simulink model "AFCSModel"  (R2025b)
settings: Solver=ode4  StartTime=0.0  StopTime=200  FixedStep=0.01  RelTol=1e-3  EnableMultiTasking=on
values from neighbouring files (symbols this model uses):
  AD = [0.05526	0.05526	0.05568	0.05804	0.06460	0.08210 ... (first row only)    [AirCraftData.m]
  Alpha0 = [0.143	0.143	0.122	-0.267	-0.627	0.120 ... (first row only)    [AirCraftData.m]
  alt = 1284.73    [Start.m]    (also in drl_simplified_dynamics.m)
  CA = 3.451    [AirCraftData.m]    (also in AircraftTrim.m)
  CDmin = [0.03799	0.03799	0.03799	0.03799	0.03904	0.04277 ... (first row only)    [AirCraftData.m]
  CLAlpha = [0.1012	0.1021	0.1033	0.1051	0.1079	0.0976 ... (first row only)    [AirCraftData.m]
  Clbt0 = [-0.00147	-0.00148	-0.00149	-0.00153	-0.00158	-0.00171 ... (first row only)    [AirCraftData.m]
  Clbtaf = [0	0	0	0	0	0;0	 0	0	0	0	0]    [AirCraftData.m]
  ClDelA = [-0.003110	-0.003065	-0.003040	-0.003036	-0.003052	-0.003088 ... (first row only)    [AirCraftData.m]
  CLDelE = [0.00653	0.00668	0.00690	0.00724	0.00772	0.00846 ... (first row only)    [AirCraftData.m]
  ClDelR = [0.000584	0.000605	0.000638	0.000686	0.000760	0.000877 ... (first row only)    [AirCraftData.m]
  CLDM = [0.244	0.244	0.244	0.244	0.244	0.244 ... (first row only)    [AirCraftData.m]
  Clp0 = [-0.5510 	-0.5610 	-0.5767 	-0.6005 	-0.6224 	-0.6763 ... (first row only)    [AirCraftData.m]
  ClpAf = [0,0,0,0,0,0;0,0,0,0,0,0]    [AirCraftData.m]
  Clr0 = [0.1308 	0.1339 	0.1383 	0.1474 	0.1601 	0.1738 ... (first row only)    [AirCraftData.m]
  ClrAf = [0,0,0,0,0,0;0,0,0,0,0,0]    [AirCraftData.m]
  Cm0 = [0.2014	0.2017	0.2034	0.2083	0.2207	0.2475 ... (first row only)    [AirCraftData.m]
  CmAfdot = [-11.5890 	-12.0169 	-12.7558 	-13.8010 	-15.2088 	-16.2278 ... (first row only)    [AirCraftData.m]
  CmCl = [-0.3454	-0.3441	-0.3427	-0.3412	-0.3396	-0.3379 ... (first row only)    [AirCraftData.m]
  CmDelE = [-0.03554	-0.03651	-0.03802	-0.04028	-0.04365	-0.04798 ... (first row only)    [AirCraftData.m]
  Cmq0 = [-42.0260 	-42.2665 	-42.9499 	-44.8315 	-45.5877 	-46.0842 ... (first row only)    [AirCraftData.m]
  CN1A0 = [0.0740	0.0662	0.0605	0.0552	0.0554 ... (first row only)    [AirCraftData.m]
  Cnbt0 = [0.00180	0.00183	0.00187	0.00192	0.00200	0.00207 ... (first row only)    [AirCraftData.m]
  Cnbtaf = [-0.000030 	-0.000031 	-0.000031 	-0.000032 	-0.000033 	-0.000035 ... (first row only)    [AirCraftData.m]
  CnDelA0 = [-0.000180	-0.000178	-0.000176	-0.000176	-0.000177	-0.000179 ... (first row only)    [AirCraftData.m]
  CnDelAAf = [0	 0	0	0	0	0;0	 0	0	0	0	0]    [AirCraftData.m]
  CnDelR = [-0.002214	-0.002274	-0.002367	-0.002505	-0.002712	-0.003039 ... (first row only)    [AirCraftData.m]
  Cnp0 = [0.0521 	0.0532 	0.0571 	0.0601 	0.0636 	0.0664 ... (first row only)    [AirCraftData.m]
  CnpAf = [0,0,0,0,0,0;0,0,0,0,0,0]    [AirCraftData.m]
  Cnr = [-0.1810 	-0.1832 	-0.1855 	-0.1892 	-0.1933 	-0.1973 ... (first row only)    [AirCraftData.m]
  Cxh_Slip = [0.0000, 0.0045, 0.0089, 0.0132, 0.0174 ... (first row only)    [AirCraftData.m]
  Cybeta0 = [-0.01783	-0.01790	-0.01804	-0.01824	-0.01851	-0.01884 ... (first row only)    [AirCraftData.m]
  Cybtaf = [0 0 0 0 0 0;0 0 0 0 0 0]    [AirCraftData.m]
  CyDelA = [0.000287	0.000295	0.000307	0.000325	0.000351	0.000394 ... (first row only)    [AirCraftData.m]
  CyDelR = [0.004946	0.005035	0.005316	0.005791	0.006458	0.007318 ... (first row only)    [AirCraftData.m]
  Cyh_Slip = [0.0000, -0.0248, -0.0519, -0.0813, -0.1130 ... (first row only)    [AirCraftData.m]
  ETA_data = [0.729 0.727 0.72 0.71 0.877 0.858 0.855 0.853 0.857 0.862 0.87 0.796 ... (330 elements, 11x5x6)]    [ETA_data.mat]
  eul_0 = [0/57.3 0/57.3 0/57.3]    [AircraftTrim.m]
  F = A(:, 1)    [drl_simplified_dynamics.m]    (also in func_DrawAircraftModel.m = [         1,  2,  3,  1;         1,  3,  4,  1;         1,  )
  flap = 0    [AircraftTrim.m]
  inertia = [  Ix      Iy     Iz  Ixz]    [AircraftTrim.m]
  Initi_Heading = 15.95*pi/180    (= 0.278380015693)    [Start.m]
  Initi_Lati = 32.6261    [Start.m]
  Initi_Longi = 103.5940    (= 103.594)    [Start.m]
  mass = 54000    [Start.m]    (also in drl_simplified_dynamics.m)
  op = evalin('base', 'op')    [drl_simplified_dynamics.m]
  q = func_GreatCircleForward(start_lat, start_lon, leg_bearing, local_s)    [system_model_update.m]
  r = r1 + r2    [drl_piecewise_reward.m]    (also in drl_reward_function.m)
  RNPAR_FlightPlan = JiuZhaiHuangLong_RNPAR_FlightPlan    [Manuscript_RNPAR_FlightPlan.m]
  Vab_0 = [Vt 0 0]    [AircraftTrim.m]
  Vt = 80    [Start.m]    (also in drl_simplified_dynamics.m; setup_afcs_system_model_test.m)
  wind_direction = 0    [Start.m]
  wind_type = 2    [Start.m]
  Wxyz_0 = [0 0 0]    [AircraftTrim.m]
  X = 1.06    [AircraftTrim.m]
  xme_0 = [0 0 -alt]    [AircraftTrim.m]
  Y = 1.177    [AircraftTrim.m]
undefined symbols (not defined in the file or in its folder): func_SystemModelMonitorBlock, Light, MIL, slselsubs, thrust_data
libraries: simulink_extras x4, aerolibatmos2 x3, aerolibconvert2 x3, aerolibwind2 x3, sharedutil x2, aerolibobsolete x1
(part 3 of 3)

== system AFCSModel/Plane&Actuator/PlaneModel/Aero Moment/Calculate pitch Moment M ==
  QS : Inport
  V alpha beta : Inport  Port=2
  delta_p : Inport  Port=3
  delta_a delta_e delta_r : Inport  Port=4
  p q r : Inport  Port=5
  Thrust : Inport  Port=6
  delta_flap : Inport  Port=7
  CA2 : Gain  Gain=CA*121.86
  CA4 : Gain  Gain=-2*(0.5208+0.5909)*9.8
  "Caculate CM " : Subsystem
  Calculate Delta_M : Subsystem
  Product4 : Product  RndMeth=Zero
  Selector13 : Selector  InputPortWidth=3  IndexOptions=Index vector (dialog)  Indices=[3]  OutputSizes=[(-2)]
  Selector2 : Selector  InputPortWidth=3  IndexOptions=Index vector (dialog)  Indices=[1 2 ]  OutputSizes=[(-2)]
  Selector3 : Selector  InputPortWidth=3  IndexOptions=Index vector (dialog)  Indices=[2]  OutputSizes=[(-2)]
  Selector9 : Selector  InputPortWidth=3  IndexOptions=Index vector (dialog)  Indices=[2]  OutputSizes=[(-2)]
  Sum4 : Sum  Inputs=++++
  disturb Moment : Gain  Gain=4*(92.12*12300+106.2*1075)*2*3.14159/60
  M : Outport
  wires:
  V alpha beta/1 -> Selector2/1
  delta_a delta_e delta_r/1 -> Selector3/1
  delta_p/1 -> "Caculate CM "/2(delta_p)
  p q r/1 -> Selector9/1, Selector13/1
  Selector9/1 -> "Caculate CM "/4(q)
  QS/1 -> CA2/1, Calculate Delta_M/2(Qs)
  CA2/1 -> Product4/1
  Product4/1 -> Sum4/1
  Thrust/1 -> CA4/1, Calculate Delta_M/3(Thrust)
  CA4/1 -> Sum4/2
  Selector13/1 -> disturb Moment/1
  disturb Moment/1 -> Sum4/4
  Sum4/1 -> M/1
  "Caculate CM "/1(Cm) -> Product4/2
  Selector3/1 -> "Caculate CM "/3(delta_e)
  Selector2/1 -> "Caculate CM "/1(" V Alpha"), Calculate Delta_M/1(" V Alpha")
  Calculate Delta_M/1(DelatM) -> Sum4/3
  delta_flap/1 -> "Caculate CM "/5(delta_flap)

== system AFCSModel/Plane&Actuator/PlaneModel/Display_Model/Normalize1 ==
  psi without normalizing : Inport
  Add6 : Sum
  Angle Conversion1 : aerolibconvert2/Angle Conversion  IU=rad  OU=deg
  Angle Conversion2 : aerolibconvert2/Angle Conversion  IU=deg  OU=rad
  Constant : Constant  Value=-360
  Constant2 : Constant  Value=360
  Constant4 : Constant  Value=360
  Math Function : Math  Operator=mod  SignedPower=on
  Math Function1 : Math  Operator=mod  SignedPower=on
  Sign : Signum
  Switch : Switch  Criteria=u2 > Threshold  SaturateOnIntegerOverflow=off  InputSameDT=off
  Switch1 : Switch  Criteria=u2 > Threshold  SaturateOnIntegerOverflow=off  InputSameDT=off
  Psi : Outport
  wires:
  Math Function/1 -> Switch1/3
  Constant2/1 -> Math Function1/2
  Math Function1/1 -> Switch1/1
  Angle Conversion1/1 -> Math Function/1, Math Function1/1, Sign/1
  Add6/1 -> Switch/3
  Switch/1 -> Angle Conversion2/1
  psi without normalizing/1 -> Angle Conversion1/1
  Constant/1 -> Math Function/2
  Constant4/1 -> Add6/2
  Sign/1 -> Switch1/2
  Switch1/1 -> Switch/1, Add6/1, Switch/2
  Angle Conversion2/1 -> Psi/1

== system AFCSModel/Plane&Actuator/PlaneModel/Display_Model/Position Caculate ==
  VE : Inport
  VN : Inport  Port=2
  H_in : Inport  Port=3
  Add{,1..3} (4 alike) : Sum
  Divide : Product  Inputs=/*
  Divide1 : Product  Inputs=*/
  Divide2 : Product  Inputs=*/
  Gain : Gain  Gain=180/pi
  Gain1 : Gain  Gain=180/pi
  Gain2 : Gain  Gain=pi/180
  Initial Latitudinal1 : Constant  Value=Initi_Longi
  Initial Latitudinal2 : Constant  Value=Initi_Lati
  Integrator : Integrator
  Integrator1 : Integrator
  Subsystem : Subsystem
  Trigonometric Function3 : Trigonometry  Operator=cos
  Latitude : Outport
  Longitude : Outport  Port=2
  wires:
  Integrator1/1 -> Add/1
  Integrator/1 -> Add1/1
  Gain2/1 -> Trigonometric Function3/1
  Gain1/1 -> Integrator/1
  Gain/1 -> Integrator1/1
  Add1/1 -> Longitude/1
  Initial Latitudinal1/1 -> Add1/2
  Divide1/1 -> Gain1/1
  Divide2/1 -> Divide1/1
  Trigonometric Function3/1 -> Divide1/2
  Add/1 -> Subsystem/1(L), Latitude/1, Gain2/1
  VN/1 -> Divide/2
  Initial Latitudinal2/1 -> Add/2
  Divide/1 -> Gain/1
  VE/1 -> Divide2/1
  Subsystem/1(RN) -> Add2/2
  H_in/1 -> Add3/2, Add2/1
  Add2/1 -> Divide2/2
  Subsystem/2(RM) -> Add3/1
  Add3/1 -> Divide/1

== system AFCSModel/Plane&Actuator/PlaneModel/Display_Model/TAS-IAS ==
  H : Inport
  V : Inport  Port=2
  TAS-EAS1 : Subsystem
  IAS : Outport
  wires:
  V/1 -> TAS-EAS1/1(TAS  (m/s))
  H/1 -> TAS-EAS1/2(Height  (m))
  TAS-EAS1/1(EAS (m/s)) -> IAS/1

== system AFCSModel/Plane&Actuator/PlaneModel/RusPlane/AV Alpha Beta ==
  udot vdot wdot : Inport
  Alpha dot : Fcn  Expr="(  - u[1]*u[6] + u[3]*u[4]  ) / ( u[4]*u[4]+ u[6]*u[6] )"
  Beta dot : Fcn  Expr="( u[7]*u[2]-u[5]*( (  u[1]*u[4] + u[2]*u[5] + u[3]*u[6] ) / u[7] ) ) / ( cos(u[9])*u[7]*u[7] )"
  Mux : Mux  Inputs=3
  Mux1 : Mux  Inputs=[3 3 3]
  Mux2 : Mux  Inputs=3
  V alpha beta : Integrator  InitialCondition=op.States(1).x
  V dot : Fcn  Expr="(  u[1]*u[4] + u[2]*u[5] + u[3]*u[6] ) / u[7]"
  "Vx " : Fcn  Expr=u[1]*cos(u[2])*cos(u[3])
  Vy1 : Fcn  Expr=u[1]*sin(u[2])*cos(u[3])
  Vz1 : Fcn  Expr=u[1]*sin(u[3])
  V alpha beta : Outport  InitialOutput=0
  u v w in : Outport  Port=2  InitialOutput=0
  wires:
  Mux2/1 -> V alpha beta/1
  V dot/1 -> Mux2/1
  Alpha dot/1 -> Mux2/2
  Beta dot/1 -> Mux2/3
  udot vdot wdot/1 -> Mux1/1
  Mux1/1 -> Alpha dot/1, V dot/1, Beta dot/1
  V alpha beta/1 -> V alpha beta/1, Mux1/3, "Vx "/1, Vz1/1, Vy1/1
  Mux/1 -> Mux1/2, u v w in/1
  "Vx "/1 -> Mux/1  "u"
  Vz1/1 -> Mux/2  "v"
  Vy1/1 -> Mux/3  "w"

== system AFCSModel/Plane&Actuator/PlaneModel/RusPlane/AV Alpha Beta_Trans ==
  V alpha beta input : Inport
  Alpha : Fcn  Expr=atan(u(3) / u(1))
  Beta : Fcn  Expr=asin(u(2) / sqrt(u(1)^2 + u(2)^2 + u(3)^2))
  Memory : Memory
  Mux : Mux  Inputs=3
  Mux2 : Mux  Inputs=3
  Sum3 : Sum  Inputs=+-
  V : Fcn  Expr=sqrt(u(1)^2 + u(2)^2 + u(3)^2)
  "Vx " : Fcn  Expr=u[1]*cos(u[2])*cos(u[3])
  Vy1 : Fcn  Expr=u[1]*sin(u[2])*cos(u[3])
  Vz1 : Fcn  Expr=u[1]*sin(u[3])
  Valphabeta : Outport
  wires:
  Vz1/1 -> Mux/2  "v"
  "Vx "/1 -> Mux/1  "u"
  Vy1/1 -> Mux/3  "w"
  V alpha beta input/1 -> Vy1/1, Vz1/1, "Vx "/1
  Mux/1 -> Sum3/1
  Mux2/1 -> Valphabeta/1
  Alpha/1 -> Mux2/2
  Beta/1 -> Mux2/3
  V/1 -> Mux2/1
  Sum3/1 -> V/1, Beta/1, Alpha/1
  [uvw_body] -> Memory/1
  Memory/1 -> Sum3/2

== system AFCSModel/Plane&Actuator/PlaneModel/RusPlane/Calculate DCM & Euler Angles ==
  "Wxyz " : Inport
  phi theta psi : Integrator  InitialCondition=[op.States(3).x(1) op.States(3).x(2) Initi_Heading]
  phidot psidot thetadot : Subsystem
  Euler : Outport
  wires:
  "Wxyz "/1 -> phidot psidot thetadot/1(Wx Wy Wz)
  phidot psidot thetadot/1(phidot thetadot psidot) -> phi theta psi/1
  phi theta psi/1 -> Euler/1, phidot psidot thetadot/2(phi theta psi)

== system AFCSModel/Plane&Actuator/PlaneModel/RusPlane/Subsystem ==
  Moment L M N : Inport
  pqr : Inport  Port=2
  inertia Ix Iy Iz Ixz : Inport  Port=3
  Beta dot : Fcn  Expr="( u[7]*u[3]+  u[1]*u[10] +  u[5]*u[6]*u[10]*(  u[8]-u[9]-u[7] )+  u[4]*u[5]*(  u[7]^2 - u[10]^2-u[7]*u[8]) ) / (u[7]*u[9]-u[10]^2)"
  Mux1 : Mux  Inputs=[3 3 4]
  Mux2 : Mux  Inputs=3
  p dot : Fcn  Expr=(u[1]*u[9] + u[3]*u[10] +u[4]*u[5]*u[10]* (u[7]+u[9]-u[8])-u[5]*u[6]*(u[9]^2+u[10]^2-u[8]*u[9])) / (u[7]*u[9]-u[10]^2)
  q dot : Fcn  Expr="( u[2]-u[4]*u[6]*(u[7]-u[9]) - u[10]*(u[4]^2-u[6]^2)  ) / u[8]"
  pdot qdot rdot : Outport
  wires:
  Mux1/1 -> Beta dot/1, p dot/1, q dot/1
  Mux2/1 -> pdot qdot rdot/1
  Beta dot/1 -> Mux2/3
  q dot/1 -> Mux2/2
  p dot/1 -> Mux2/1
  inertia Ix Iy Iz Ixz/1 -> Mux1/3
  pqr/1 -> Mux1/2
  Moment L M N/1 -> Mux1/1

== system AFCSModel/Plane&Actuator/PlaneModel/RusPlane/Subsystem1 ==
  "U V W " : Inport
  Euler phi theta psi : Inport  Port=2
  Mux1 : Mux  Inputs=[3 3 ]
  Mux2 : Mux  Inputs=3
  Xe dot : Fcn  Expr="u[1]*cos(u[5])*cos(u[6])  +   u[2]*(sin(u[4])*sin(u[5]) *cos(u[6])-cos(u[4])*sin(u[6]) )  +u[3]*(sin(u[4])*sin(u[6])+cos(u[4])*sin(u[5])*cos(u[6])  )"
  Ye dot : Fcn  Expr="u[1]*cos(u[5])*sin(u[6])  + u[2]*(sin(u[4])*sin(u[5])*sin(u[6]) + cos(u[4])*cos(u[6]) )  + u[3]*( cos(u[4])*sin(u[5])*sin(u[6])-sin(u[4])*cos(u[6]) )"
  Ze dot : Fcn  Expr="u[2]*sin(u[4])*cos(u[5])  + u[3]*cos(u[4])*cos(u[5]) -u[1]*sin(u[5])"
  Xedot Yedot Zedot : Outport
  wires:
  Xe dot/1 -> Mux2/1
  Ze dot/1 -> Mux2/3
  Mux2/1 -> Xedot Yedot Zedot/1
  "U V W "/1 -> Mux1/1
  Euler phi theta psi/1 -> Mux1/2
  Mux1/1 -> Xe dot/1, Ye dot/1, Ze dot/1
  Ye dot/1 -> Mux2/2

== system AFCSModel/Plane&Actuator/PlaneModel/Aero Force/Caculate Y/Cy_beta ==
  Ma : Inport
  alpha : Inport  Port=2
  delta_flap : Inport  Port=3
  Add1 : Sum
  Cy_beta0 : Lookup2D  RowIndex=[0 6/57.3]  ColumnIndex=Mach_table  Table=Cybeta0  SaturateOnIntegerOverflow=off  InputSameDT=off
  Cy_beta_alpha : Lookup2D  RowIndex=[0 6/57.3]  ColumnIndex=Mach_table  Table=Cybtaf  SaturateOnIntegerOverflow=off  InputSameDT=off
  Product5 : Product  RndMeth=Zero
  Cybeta : Outport
  wires:
  Cy_beta0/1 -> Add1/1
  Cy_beta_alpha/1 -> Product5/1
  Product5/1 -> Add1/2
  Ma/1 -> Cy_beta0/2, Cy_beta_alpha/2
  Add1/1 -> Cybeta/1
  alpha/1 -> Product5/2
  delta_flap/1 -> Cy_beta0/1, Cy_beta_alpha/1

== system AFCSModel/Plane&Actuator/PlaneModel/Aero Force/Calculate  Lift/Caculate CL ==
  Alpha : Inport
  delta_e : Inport  Port=2
  delta_flap : Inport  Port=3
  Alpha_0 : Lookup2D  RowIndex=[0 6/57.3]  ColumnIndex=Mach_table  Table=Alpha0  SaturateOnIntegerOverflow=off  InputSameDT=off
  Cl_alpha : Lookup2D  RowIndex=[0 6/57.3]  ColumnIndex=Mach_table  Table=CLAlpha  SaturateOnIntegerOverflow=off  InputSameDT=off
  Cl_alpha*alpha : Product  RndMeth=Zero
  Cl_delta_e*delta_e : Product  RndMeth=Zero
  Cldelta_e : Lookup2D  RowIndex=[0 6/57.3]  ColumnIndex=Mach_table  Table=CLDelE  SaturateOnIntegerOverflow=off  InputSameDT=off
  Constant : Constant  Value=4/57.3
  Subtract : Sum
  Subtract1 : Sum  Inputs=+-
  Subtract2 : Sum
  CL : Outport
  wires:
  Cldelta_e/1 -> Cl_delta_e*delta_e/1
  delta_e/1 -> Cl_delta_e*delta_e/2
  Constant/1 -> Subtract/1
  Alpha/1 -> Subtract/2
  [Ma] -> Alpha_0/2, Cldelta_e/2, Cl_alpha/2
  Subtract/1 -> Subtract1/1
  Alpha_0/1 -> Subtract1/2
  Cl_alpha/1 -> Cl_alpha*alpha/1
  Subtract1/1 -> Cl_alpha*alpha/2
  Cl_alpha*alpha/1 -> Subtract2/1
  Cl_delta_e*delta_e/1 -> Subtract2/2
  Subtract2/1 -> CL/1
  delta_flap/1 -> Cl_alpha/1, Alpha_0/1, Cldelta_e/1

== system AFCSModel/Plane&Actuator/PlaneModel/Aero Force/Calculate  Lift/SlipStream Strength B ==
  Thrust : Inport
  Qs : Inport  Port=2
  Divide : Product  Inputs=*/
  S : Gain  Gain=12.566
  B : Outport
  wires:
  S/1 -> Divide/2
  Qs/1 -> S/1
  Divide/1 -> B/1
  Thrust/1 -> Divide/1

== system AFCSModel/Plane&Actuator/PlaneModel/Aero Force/Calculate  Lift/alpha_w_deg ==
  In1 : Inport
  Constant : Constant  Value=4
  S3 : Gain  Gain=57.3
  Subtract : Sum
  Out1 : Outport
  wires:
  S3/1 -> Subtract/1
  Constant/1 -> Subtract/2
  In1/1 -> S3/1
  Subtract/1 -> Out1/1

== system AFCSModel/Plane&Actuator/PlaneModel/Aero Force/Calculate Drag/Caculate CD  ==
  " delta_flap" : Inport
  "  Alpha_w" : Inport  Port=2
  AD : Lookup2D  RowIndex=[0 6/57.3]  ColumnIndex=Mach_table  Table=AD  SaturateOnIntegerOverflow=off  InputSameDT=off
  Add : Sum
  Alpha0 : Lookup2D  RowIndex=[0 6/57.3]  ColumnIndex=Mach_table  Table=Alpha0  SaturateOnIntegerOverflow=off  InputSameDT=off
  CDmin : Lookup2D  RowIndex=[0 6/57.3]  ColumnIndex=Mach_table  Table=CDmin  SaturateOnIntegerOverflow=off  InputSameDT=off
  CLDM : Lookup2D  RowIndex=[0 6/57.3]  ColumnIndex=Mach_table  Table=CLDM  SaturateOnIntegerOverflow=off  InputSameDT=off
  Cl_alpha : Lookup2D  RowIndex=[0 6/57.3]  ColumnIndex=Mach_table  Table=CLAlpha  SaturateOnIntegerOverflow=off  InputSameDT=off
  Product : Product  RndMeth=Zero
  Product1 : Product  RndMeth=Zero
  Product2 : Product  RndMeth=Zero
  Subtract : Sum  Inputs=+-
  alpha_w-alpha0 : Sum  Inputs=-+
  CD : Outport
  wires:
  [Ma] -> Alpha0/2, CLDM/2, Cl_alpha/2, AD/2, CDmin/2
  CDmin/1 -> Add/1
  "  Alpha_w"/1 -> alpha_w-alpha0/2
  Alpha0/1 -> alpha_w-alpha0/1
  alpha_w-alpha0/1 -> Product/2
  Cl_alpha/1 -> Product/1
  Product/1 -> Subtract/1
  CLDM/1 -> Subtract/2
  Subtract/1 -> Product1/1, Product1/2
  AD/1 -> Product2/1
  Product1/1 -> Product2/2
  Product2/1 -> Add/2
  Add/1 -> CD/1
  " delta_flap"/1 -> CDmin/1, AD/1, Cl_alpha/1, Alpha0/1, CLDM/1

== system AFCSModel/Plane&Actuator/PlaneModel/Aero Force/Calculate Drag/SlipStream Strength B ==
  Thrust : Inport
  Qs : Inport  Port=2
  Divide : Product  Inputs=*/
  S : Gain  Gain=12.566
  B : Outport
  wires:
  S/1 -> Divide/2
  Qs/1 -> S/1
  Divide/1 -> B/1
  Thrust/1 -> Divide/1

== system AFCSModel/Plane&Actuator/PlaneModel/Aero Force/Calculate Drag/alpha_w_deg ==
  In1 : Inport
  Constant : Constant  Value=4
  S3 : Gain  Gain=57.3
  Subtract : Sum
  Out1 : Outport
  wires:
  S3/1 -> Subtract/1
  Constant/1 -> Subtract/2
  In1/1 -> S3/1
  Subtract/1 -> Out1/1

== system AFCSModel/Plane&Actuator/PlaneModel/Aero Moment/Calculate Roll Moment L/airdata ==
  V Alpha Beta : Inport
  delta_p : Inport  Port=2
  delta_flap : Inport  Port=3
  Add : Sum
  CN_alpha : Subsystem
  Cl_beta : Subsystem
  Cl_beta* : Sum
  Cl_delta_a : Lookup2D  RowIndex=[0 6/57.3]  ColumnIndex=Mach_table  Table=ClDelA  SaturateOnIntegerOverflow=off  InputSameDT=off
  Cl_delta_r : Lookup2D  RowIndex=[0 6/57.3]  ColumnIndex=Mach_table  Table=ClDelR  SaturateOnIntegerOverflow=off  InputSameDT=off
  Cl_delta_r* : Sum
  Cl_p : Subsystem
  Cl_r : Subsystem
  Cy_beta : Subsystem
  Cy_delta_r : Lookup2D  RowIndex=[0 6/57.3]  ColumnIndex=Mach_table  Table=CyDelR  SaturateOnIntegerOverflow=off  InputSameDT=off
  Gain : Gain  Gain=(Y-0.85)/38
  Gain1 : Gain  Gain=(Y-0.85)/38
  Mux2 : Mux  Inputs=5
  Selector1 : Selector  InputPortWidth=3  IndexOptions=Index vector (dialog)  Indices=[2]  OutputSizes=[(-2)]
  Selector12 : Selector  InputPortWidth=3  IndexOptions=Index vector (dialog)  Indices=[2]  OutputSizes=[(-2)]
  Cl_beta Cl_delta_a Cl_delta_r Cl_p Cl_r : Outport
  wires:
  [Ma] -> Cl_p/2(Ma), Cl_r/2(Ma), Cy_delta_r/2, Cl_delta_r/2, Cl_delta_a/2, Cy_beta/3(Ma), Cl_beta/1(Ma)
  Mux2/1 -> Cl_beta Cl_delta_a Cl_delta_r Cl_p Cl_r/1
  delta_p/1 -> CN_alpha/2(delta_p)
  V Alpha Beta/1 -> CN_alpha/1(V), Selector12/1, Selector1/1
  CN_alpha/1(Out1) -> Add/2
  Cy_beta/1(Cybeta) -> Gain/1
  Gain/1 -> Cl_beta*/2
  Add/1 -> Cl_beta*/1
  Cy_delta_r/1 -> Gain1/1
  Cl_delta_r/1 -> Cl_delta_r*/1
  Gain1/1 -> Cl_delta_r*/2
  Cl_beta*/1 -> Mux2/1
  Cl_delta_a/1 -> Mux2/2
  Cl_delta_r*/1 -> Mux2/3
  Cl_p/1(Cl_p) -> Mux2/4
  Cl_r/1(Cl_r) -> Mux2/5
  Selector12/1 -> Cl_p/1(alpha), Cl_r/1(alpha), Cl_r/3(delta_flap), Cy_beta/1(alpha)
  Cl_beta/1(C1beta) -> Add/1
  Selector1/1 -> Cl_beta/2(alpha)
  delta_flap/1 -> Cl_beta/3(delta_flap), Cy_beta/2(delta_flap), Cl_delta_a/1, Cl_delta_r/1, Cy_delta_r/1, Cl_p/3(delta_flap)

== system AFCSModel/Plane&Actuator/PlaneModel/Aero Moment/Calculate Yaw Moment N/aeroMoment coef ==
  V Alpha Beta : Inport
  delta_p : Inport  Port=2
  delta_flap : Inport  Port=3
  CN_alpha : Subsystem
  Cn_beta : Subsystem
  Cn_beta* : Sum  Inputs=+++
  Cn_delta_a1 : Subsystem
  Cn_delta_r : Lookup2D  RowIndex=[0 6/57.3]  ColumnIndex=Mach_table  Table=CnDelR  SaturateOnIntegerOverflow=off  InputSameDT=off
  Cn_delta_r* : Sum
  Cn_p : Subsystem
  Cn_r : Lookup2D  RowIndex=[0 6/57.3]  ColumnIndex=Mach_table  Table=Cnr  SaturateOnIntegerOverflow=off  InputSameDT=off
  Cy_beta : Subsystem
  Cy_delta_r : Lookup2D  RowIndex=[0 6/57.3]  ColumnIndex=Mach_table  Table=CyDelR  SaturateOnIntegerOverflow=off  InputSameDT=off
  Gain : Gain  Gain=(X-1.036514)/38
  Gain1 : Gain  Gain=(X-1.036514)/38
  Mux2 : Mux  Inputs=5
  Selector1 : Selector  InputPortWidth=3  IndexOptions=Index vector (dialog)  Indices=[1]  OutputSizes=[(-2)]
  Selector12 : Selector  InputPortWidth=3  IndexOptions=Index vector (dialog)  Indices=[2]  OutputSizes=[(-2)]
  Cn_beta Cn_delta_r Cl_delta_a Cn_p Cn_r : Outport
  wires:
  [Ma] -> Cn_p/2(Ma), Cn_r/2, Cn_delta_a1/2(Ma), Cy_delta_r/2, Cn_delta_r/2, Cy_beta/2(Ma), Cn_beta/2(Ma)
  Mux2/1 -> Cn_beta Cn_delta_r Cl_delta_a Cn_p Cn_r/1
  delta_p/1 -> CN_alpha/2(delta_p)
  V Alpha Beta/1 -> Selector12/1, Selector1/1
  Cn_beta*/1 -> Mux2/1
  CN_alpha/1(Out1) -> Cn_beta*/1
  Cn_beta/1(Cnbeta) -> Cn_beta*/2
  Cy_beta/1(Cybeta) -> Gain/1
  Gain/1 -> Cn_beta*/3
  Cy_delta_r/1 -> Gain1/1
  Gain1/1 -> Cn_delta_r*/2
  Cn_delta_r/1 -> Cn_delta_r*/1
  Cn_delta_r*/1 -> Mux2/2
  Cn_delta_a1/1(Cn_delta_a) -> Mux2/3
  Cn_p/1(Cn_p) -> Mux2/4
  Cn_r/1 -> Mux2/5
  Selector12/1 -> Cn_beta/1(alpha), Cy_beta/1(alpha), Cn_delta_a1/1(alpha), Cn_p/1(alpha)
  Selector1/1 -> CN_alpha/1(V)
  delta_flap/1 -> Cn_beta/3(delta_flap), Cy_beta/3(delta_flap), Cn_delta_r/1, Cy_delta_r/1, Cn_delta_a1/3(delta_flap), Cn_p/3(delta_flap), Cn_r/1

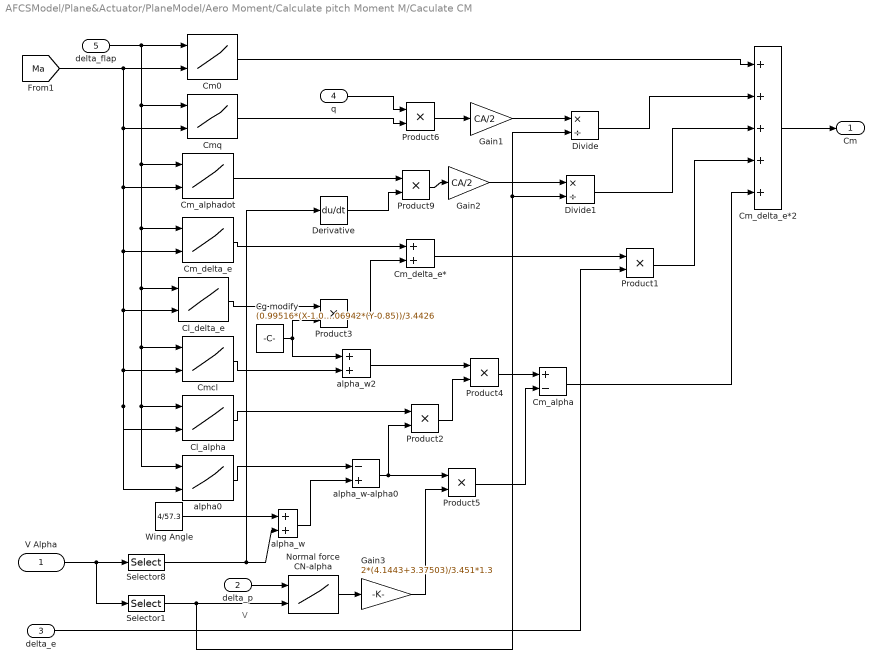
== system AFCSModel/Plane&Actuator/PlaneModel/Aero Moment/Calculate pitch Moment M/Caculate CM  ==
  note: V
  " V Alpha" : Inport
  delta_p : Inport  Port=2
  delta_e : Inport  Port=3
  q : Inport  Port=4
  delta_flap : Inport  Port=5
  Cg modify : Constant  Value=(0.99516*(X-1.036514)-0.06942*(Y-0.85))/3.4426
  Cl_alpha : Lookup2D  RowIndex=[0 6/57.3]  ColumnIndex=Mach_table  Table=CLAlpha  SaturateOnIntegerOverflow=off  InputSameDT=off
  Cl_delta_e : Lookup2D  RowIndex=[0 6/57.3]  ColumnIndex=Mach_table  Table=CLDelE  SaturateOnIntegerOverflow=off  InputSameDT=off
  Cm0 : Lookup2D  RowIndex=[0 6/57.3]  ColumnIndex=Mach_table  Table=Cm0  SaturateOnIntegerOverflow=off  InputSameDT=off
  Cm_alpha : Sum  Inputs=+-
  Cm_alphadot : Lookup2D  RowIndex=[0 6/57.3]  ColumnIndex=Mach_table  Table=CmAfdot  SaturateOnIntegerOverflow=off  InputSameDT=off
  Cm_delta_e : Lookup2D  RowIndex=[0 6/57.3]  ColumnIndex=Mach_table  Table=CmDelE  SaturateOnIntegerOverflow=off  InputSameDT=off
  Cm_delta_e* : Sum
  Cm_delta_e*2 : Sum  Inputs=+++++
  Cmcl : Lookup2D  RowIndex=[0 6/57.3]  ColumnIndex=Mach_table  Table=CmCl  SaturateOnIntegerOverflow=off  InputSameDT=off
  Cmq : Lookup2D  RowIndex=[0 6/57.3]  ColumnIndex=Mach_table  Table=Cmq0  SaturateOnIntegerOverflow=off  InputSameDT=off
  Derivative : Derivative
  Divide : Product  Inputs=*/
  Divide1 : Product  Inputs=*/
  Gain1 : Gain  Gain=CA/2
  Gain2 : Gain  Gain=CA/2
  Gain3 : Gain  Gain=2*(4.1443+3.37503)/3.451*1.3
  Normal force CN-alpha : Lookup2D  RowIndex=[0.4,0.7,0.85,1,1.04]  ColumnIndex=[50,75,100,150,175]  Table=CN1A0  SaturateOnIntegerOverflow=off  InputSameDT=off
  Product{1..6,9} (7 alike) : Product  RndMeth=Zero
  Selector1 : Selector  InputPortWidth=2  IndexOptions=Index vector (dialog)  Indices=[1]  OutputSizes=[(-2)]
  Selector8 : Selector  InputPortWidth=2  IndexOptions=Index vector (dialog)  Indices=[2]  OutputSizes=[(-2)]
  Wing Angle : Constant  Value=4/57.3
  alpha0 : Lookup2D  RowIndex=[0 6/57.3]  ColumnIndex=Mach_table  Table=Alpha0  SaturateOnIntegerOverflow=off  InputSameDT=off
  alpha_w : Sum
  alpha_w-alpha0 : Sum  Inputs=-+
  alpha_w2 : Sum
  Cm : Outport
  wires:
  [Ma] -> Cl_alpha/2, alpha0/2, Cmcl/2, Cl_delta_e/2, Cm_delta_e/2, Cm_alphadot/2, Cmq/2, Cm0/2
  Cm_delta_e*2/1 -> Cm/1
  " V Alpha"/1 -> Selector8/1, Selector1/1
  Wing Angle/1 -> alpha_w/1
  Selector8/1 -> alpha_w/2, Derivative/1
  alpha0/1 -> alpha_w-alpha0/1
  alpha_w/1 -> alpha_w-alpha0/2
  alpha_w-alpha0/1 -> Product2/2, Product5/1
  Cl_alpha/1 -> Product2/1
  Normal force CN-alpha/1 -> Gain3/1
  Selector1/1 -> Divide/2, Divide1/2, Normal force CN-alpha/2
  alpha_w2/1 -> Product4/1
  Cg modify/1 -> Product3/2, alpha_w2/1
  Cl_delta_e/1 -> Product3/1
  Cm_delta_e/1 -> Cm_delta_e*/1
  Product3/1 -> Cm_delta_e*/2
  Product2/1 -> Product4/2
  Product4/1 -> Cm_alpha/1
  Gain3/1 -> Product5/2
  Product5/1 -> Cm_alpha/2
  Cmcl/1 -> alpha_w2/2
  delta_e/1 -> Product1/2
  Cm_delta_e*/1 -> Product1/1
  q/1 -> Product6/1
  Cmq/1 -> Product6/2
  Product6/1 -> Gain1/1
  Gain1/1 -> Divide/1
  Gain2/1 -> Divide1/1
  Product9/1 -> Gain2/1
  Derivative/1 -> Product9/2
  Cm_alphadot/1 -> Product9/1
  Cm0/1 -> Cm_delta_e*2/1
  Divide/1 -> Cm_delta_e*2/2
  Divide1/1 -> Cm_delta_e*2/3
  Product1/1 -> Cm_delta_e*2/4
  Cm_alpha/1 -> Cm_delta_e*2/5
  delta_p/1 -> Normal force CN-alpha/1
  delta_flap/1 -> Cm0/1, Cmq/1, Cm_alphadot/1, Cm_delta_e/1, Cl_delta_e/1, Cmcl/1, Cl_alpha/1, alpha0/1

== system AFCSModel/Plane&Actuator/PlaneModel/Aero Moment/Calculate pitch Moment M/Calculate Delta_M ==
  " V Alpha" : Inport
  Qs : Inport  Port=2
  Thrust : Inport  Port=3
  Add : Sum  Inputs=+-
  Add1 : Sum
  Add2 : Sum  Inputs=+-
  Divide : Product  Inputs=*/
  S : Gain  Gain=121.86
  S1 : Gain  Gain=2*(1.1903+1.1465)
  S2 : Gain  Gain=12.566
  S3 : Gain  Gain=1/4
  S4 : Gain  Gain=1/4
  Selector8 : Selector  InputPortWidth=2  IndexOptions=Index vector (dialog)  Indices=[2]  OutputSizes=[(-2)]
  Slipstream CD : Lookup2D  RowIndex=[0,2,4,6,8,10,12,14,16,18]  ColumnIndex=[0,0.25,0.5,0.75,1]  Table=Cxh_Slip  SaturateOnIntegerOverflow=off  InputSameDT=off
  Slipstream CL : Lookup2D  RowIndex=[0,2,4,6,8,10,12,14,16 18]  ColumnIndex=[0 0.25 0.5 0.75 1]  Table=Cyh_Slip  SaturateOnIntegerOverflow=off  InputSameDT=off
  Trigonometric Function : Trigonometry
  X : Gain  Gain=2*(-0.15845+0.42122)
  alpha_w_deg : Subsystem
  d{,1..4} (5 alike) : Product  RndMeth=Zero
  sin alpha : Trigonometry  Operator=cos
  DelatM : Outport
  wires:
  Selector8/1 -> alpha_w_deg/1(In1), sin alpha/1, Trigonometric Function/1
  Qs/1 -> d4/2, S2/1
  Slipstream CL/1 -> S3/1
  sin alpha/1 -> d/1, d3/1
  d/1 -> Add1/1
  Add1/1 -> X/1
  Slipstream CD/1 -> S4/1
  Trigonometric Function/1 -> d1/1, d2/1
  d1/1 -> Add1/2
  X/1 -> Add/1
  S1/1 -> Add/2
  d2/1 -> Add2/1
  d3/1 -> Add2/2
  Add2/1 -> S1/1
  Add/1 -> d4/1
  d4/1 -> S/1
  S/1 -> DelatM/1
  " V Alpha"/1 -> Selector8/1
  S2/1 -> Divide/2
  Thrust/1 -> Divide/1
  Divide/1 -> Slipstream CL/2, Slipstream CD/2
  alpha_w_deg/1(Out1) -> Slipstream CL/1, Slipstream CD/1
  S3/1 -> d/2, d2/2
  S4/1 -> d1/2, d3/2

== system AFCSModel/Plane&Actuator/PlaneModel/Display_Model/Position Caculate/Subsystem ==
  L : Inport
  (1-e)^1 : Constant  Value=(2-1/298.257)*1/298.257
  1 : Constant
  2 : Constant  Value=-1.5
  3 : Constant  Value=-0.5
  Add : Sum  Inputs=+-
  Gain : Gain  Gain=1/57.3
  Math Function : Math  Operator=pow  SignedPower=on
  Math Function1 : Math  Operator=pow  SignedPower=on
  Re : Constant  Value=6378137
  Re(1-e)^2 : Constant  Value=6378137*(1-1/298.257)^2
  Trigonometric Function : Trigonometry
  VE{,1..3} (4 alike) : Product  RndMeth=Zero
  RN : Outport
  RM : Outport  Port=2
  wires:
  Gain/1 -> Trigonometric Function/1
  VE3/1 -> RN/1
  Re/1 -> VE3/2
  Math Function1/1 -> VE3/1
  3/1 -> Math Function1/2
  Math Function/1 -> VE/2
  Re(1-e)^2/1 -> VE/1
  VE/1 -> RM/1
  2/1 -> Math Function/2
  Add/1 -> Math Function1/1, Math Function/1
  VE1/1 -> Add/2
  VE2/1 -> VE1/2
  Trigonometric Function/1 -> VE2/2, VE2/1
  L/1 -> Gain/1
  (1-e)^1/1 -> VE1/1
  1/1 -> Add/1

== system AFCSModel/Plane&Actuator/PlaneModel/Display_Model/TAS-IAS/TAS-EAS1 ==
  TAS  (m/s) : Inport
  Height  (m) : Inport  Port=2
  Display1 : Display
  Divide : Product  Inputs=*/
  Fcn : Fcn  Expr=sqrt(u)
  ISA Atmosphere Model2 : aerolibatmos2/ISA Atmosphere Model  useExtended=off  action=Warning  custom=off  viscosityOut=off  g=9.80665  gamma=1.4  R=287.0531  L=0.0065  h_trop=11000  h_strat=20000  rho0=1.225  P0=101325  T0=288.15  h0=0  S=110.4  Tref=273.15  muref=1.716e-5
  Product : Product  RndMeth=Zero
  Rou_o : Constant  Value=1.225
  Terminator : Terminator
  Terminator1 : Terminator
  Terminator2 : Terminator
  EAS (m/s) : Outport
  wires:
  TAS  (m/s)/1 -> Product/2
  Fcn/1 -> Product/1
  ISA Atmosphere Model2/3 -> Terminator2/1
  ISA Atmosphere Model2/2 -> Terminator1/1
  ISA Atmosphere Model2/1 -> Terminator/1
  Product/1 -> EAS (m/s)/1, Display1/1
  Divide/1 -> Fcn/1
  ISA Atmosphere Model2/4 -> Divide/1
  Height  (m)/1 -> ISA Atmosphere Model2/1
  Rou_o/1 -> Divide/2

== system AFCSModel/Plane&Actuator/PlaneModel/RusPlane/Calculate DCM & Euler Angles/phidot psidot thetadot ==
  note: p
      | q
      | r
  Wx Wy Wz : Inport
  phi theta psi : Inport  Port=2
  Mux1 : Mux  Inputs=[3 3 3]
  Mux2 : Mux  Inputs=3
  SinCos : aerolibobsolete/SinCos
  phidot : Fcn  Expr=u[1]+(u[2]*u[4]+u[3]*u[7])*(u[5]/u[8])
  psidot : Fcn  Expr=(u[2]*u[4]+u[3]*u[7])/u[8]
  thetadot : Fcn  Expr=u[2]*u[7]-u[3]*u[4]
  phidot thetadot psidot : Outport  InitialOutput=0
  wires:
  SinCos/2 -> Mux1/3
  SinCos/1 -> Mux1/2
  Mux2/1 -> phidot thetadot psidot/1
  phidot/1 -> Mux2/1
  thetadot/1 -> Mux2/2
  psidot/1 -> Mux2/3
  phi theta psi/1 -> SinCos/1
  Wx Wy Wz/1 -> Mux1/1
  Mux1/1 -> thetadot/1, phidot/1, psidot/1

== system AFCSModel/Plane&Actuator/PlaneModel/Aero Moment/Calculate Roll Moment L/airdata/CN_alpha ==
  V : Inport
  delta_p : Inport  Port=2
  Gain3 : Gain  Gain=2*(0.5208+0.5909)/38
  Normal force CN-alpha : Lookup2D  RowIndex=[0.4,0.7,0.85,1,1.04]  ColumnIndex=[50,75,100,150,175]  Table=CN1A0  SaturateOnIntegerOverflow=off  InputSameDT=off
  Selector12 : Selector  InputPortWidth=3  IndexOptions=Index vector (dialog)  Indices=[1]  OutputSizes=[(-2)]
  Out1 : Outport
  wires:
  Normal force CN-alpha/1 -> Gain3/1
  V/1 -> Selector12/1
  Gain3/1 -> Out1/1
  delta_p/1 -> Normal force CN-alpha/1
  Selector12/1 -> Normal force CN-alpha/2

== system AFCSModel/Plane&Actuator/PlaneModel/Aero Moment/Calculate Roll Moment L/airdata/Cl_beta ==
  Ma : Inport
  alpha : Inport  Port=2
  delta_flap : Inport  Port=3
  Add1 : Sum
  Cl_beta0 : Lookup2D  RowIndex=[0 6/57.3]  ColumnIndex=Mach_table  Table=Clbt0  SaturateOnIntegerOverflow=off  InputSameDT=off
  Cl_beta_alpha : Lookup2D  RowIndex=[0 6/57.3]  ColumnIndex=Mach_table  Table=Clbtaf  SaturateOnIntegerOverflow=off  InputSameDT=off
  Product5 : Product  RndMeth=Zero
  C1beta : Outport
  wires:
  Cl_beta0/1 -> Add1/1
  Cl_beta_alpha/1 -> Product5/1
  Product5/1 -> Add1/2
  Ma/1 -> Cl_beta0/2, Cl_beta_alpha/2
  Add1/1 -> C1beta/1
  alpha/1 -> Product5/2
  delta_flap/1 -> Cl_beta0/1, Cl_beta_alpha/1

== system AFCSModel/Plane&Actuator/PlaneModel/Aero Moment/Calculate Roll Moment L/airdata/Cl_p ==
  alpha : Inport
  Ma : Inport  Port=2
  delta_flap : Inport  Port=3
  Add1 : Sum
  Cl_p0 : Lookup2D  RowIndex=[0 6/57.3]  ColumnIndex=Mach_table  Table=Clp0  SaturateOnIntegerOverflow=off  InputSameDT=off
  Clp_alpha : Lookup2D  RowIndex=[0 6/57.3]  ColumnIndex=Mach_table  Table=ClpAf  SaturateOnIntegerOverflow=off  InputSameDT=off
  Product5 : Product  RndMeth=Zero
  Cl_p : Outport
  wires:
  alpha/1 -> Product5/2
  Add1/1 -> Cl_p/1
  Ma/1 -> Cl_p0/2, Clp_alpha/2
  Product5/1 -> Add1/2
  Clp_alpha/1 -> Product5/1
  Cl_p0/1 -> Add1/1
  delta_flap/1 -> Cl_p0/1, Clp_alpha/1

== system AFCSModel/Plane&Actuator/PlaneModel/Aero Moment/Calculate Roll Moment L/airdata/Cl_r ==
  alpha : Inport
  Ma : Inport  Port=2
  delta_flap : Inport  Port=3
  Add1 : Sum
  Cl_r0 : Lookup2D  RowIndex=[0 6/57.3]  ColumnIndex=Mach_table  Table=Clr0  SaturateOnIntegerOverflow=off  InputSameDT=off
  Clr_alpha : Lookup2D  RowIndex=[0 6/57.3]  ColumnIndex=Mach_table  Table=ClrAf  SaturateOnIntegerOverflow=off  InputSameDT=off
  Product5 : Product  RndMeth=Zero
  Cl_r : Outport
  wires:
  Cl_r0/1 -> Add1/1
  Clr_alpha/1 -> Product5/1
  Product5/1 -> Add1/2
  Ma/1 -> Cl_r0/2, Clr_alpha/2
  Add1/1 -> Cl_r/1
  alpha/1 -> Product5/2
  delta_flap/1 -> Cl_r0/1, Clr_alpha/1

== system AFCSModel/Plane&Actuator/PlaneModel/Aero Moment/Calculate Roll Moment L/airdata/Cy_beta ==
  alpha : Inport
  delta_flap : Inport  Port=2
  Ma : Inport  Port=3
  Add1 : Sum
  Cy_beta0 : Lookup2D  RowIndex=[0 6/57.3]  ColumnIndex=Mach_table  Table=Cybeta0  SaturateOnIntegerOverflow=off  InputSameDT=off
  Cy_beta_alpha : Lookup2D  RowIndex=[0 6/57.3]  ColumnIndex=Mach_table  Table=Cybtaf  SaturateOnIntegerOverflow=off  InputSameDT=off
  Product5 : Product  RndMeth=Zero
  Cybeta : Outport
  wires:
  Cy_beta0/1 -> Add1/1
  Cy_beta_alpha/1 -> Product5/1
  Product5/1 -> Add1/2
  Ma/1 -> Cy_beta0/2, Cy_beta_alpha/2
  Add1/1 -> Cybeta/1
  alpha/1 -> Product5/2
  delta_flap/1 -> Cy_beta0/1, Cy_beta_alpha/1

== system AFCSModel/Plane&Actuator/PlaneModel/Aero Moment/Calculate Yaw Moment N/aeroMoment coef/CN_alpha ==
  V : Inport
  delta_p : Inport  Port=2
  Gain3 : Gain  Gain=-2*(4.1443+3.37503)/38
  Normal force CN-alpha : Lookup2D  RowIndex=[0.4,0.7,0.85,1,1.04]  ColumnIndex=[50,75,100,150,175]  Table=CN1A0  SaturateOnIntegerOverflow=off  InputSameDT=off
  Out1 : Outport
  wires:
  Normal force CN-alpha/1 -> Gain3/1
  Gain3/1 -> Out1/1
  delta_p/1 -> Normal force CN-alpha/1
  V/1 -> Normal force CN-alpha/2

== system AFCSModel/Plane&Actuator/PlaneModel/Aero Moment/Calculate Yaw Moment N/aeroMoment coef/Cn_beta ==
  alpha : Inport
  Ma : Inport  Port=2
  delta_flap : Inport  Port=3
  Add1 : Sum
  Add2 : Sum  Inputs=+-
  Cn_beta0 : Lookup2D  RowIndex=[0 6/57.3]  ColumnIndex=Mach_table  Table=Cnbt0  SaturateOnIntegerOverflow=off  InputSameDT=off
  Cn_beta_alpha : Lookup2D  RowIndex=[0 6/57.3]  ColumnIndex=Mach_table  Table=Cnbtaf  SaturateOnIntegerOverflow=off  InputSameDT=off
  Constant : Constant  Value=4/57.3
  Product5 : Product  RndMeth=Zero
  Cnbeta : Outport
  wires:
  Add1/1 -> Cnbeta/1
  Ma/1 -> Cn_beta0/2, Cn_beta_alpha/2
  Product5/1 -> Add1/2
  Cn_beta_alpha/1 -> Product5/1
  Cn_beta0/1 -> Add1/1
  delta_flap/1 -> Cn_beta0/1, Cn_beta_alpha/1
  alpha/1 -> Add2/1
  Add2/1 -> Product5/2
  Constant/1 -> Add2/2

== system AFCSModel/Plane&Actuator/PlaneModel/Aero Moment/Calculate Yaw Moment N/aeroMoment coef/Cn_delta_a1 ==
  alpha : Inport
  Ma : Inport  Port=2
  delta_flap : Inport  Port=3
  Add1 : Sum
  Cn_delta_a0 : Lookup2D  RowIndex=[0 6/57.3]  ColumnIndex=Mach_table  Table=CnDelA0  SaturateOnIntegerOverflow=off  InputSameDT=off
  Cn_delta_alpha : Lookup2D  RowIndex=[0 6/57.3]  ColumnIndex=Mach_table  Table=CnDelAAf  SaturateOnIntegerOverflow=off  InputSameDT=off
  Product5 : Product  RndMeth=Zero
  Cn_delta_a : Outport
  wires:
  Cn_delta_a0/1 -> Add1/1
  Cn_delta_alpha/1 -> Product5/1
  Product5/1 -> Add1/2
  Ma/1 -> Cn_delta_a0/2, Cn_delta_alpha/2
  Add1/1 -> Cn_delta_a/1
  alpha/1 -> Product5/2
  delta_flap/1 -> Cn_delta_a0/1, Cn_delta_alpha/1

== system AFCSModel/Plane&Actuator/PlaneModel/Aero Moment/Calculate Yaw Moment N/aeroMoment coef/Cn_p ==
  alpha : Inport
  Ma : Inport  Port=2
  delta_flap : Inport  Port=3
  Add1 : Sum
  Cn_p0 : Lookup2D  RowIndex=[0 6/57.3]  ColumnIndex=Mach_table  Table=Cnp0  SaturateOnIntegerOverflow=off  InputSameDT=off
  Cnp_alpha : Lookup2D  RowIndex=[0 6/57.3]  ColumnIndex=Mach_table  Table=CnpAf  SaturateOnIntegerOverflow=off  InputSameDT=off
  Product5 : Product  RndMeth=Zero
  Cn_p : Outport
  wires:
  alpha/1 -> Product5/2
  Add1/1 -> Cn_p/1
  Ma/1 -> Cn_p0/2, Cnp_alpha/2
  Product5/1 -> Add1/2
  Cnp_alpha/1 -> Product5/1
  Cn_p0/1 -> Add1/1
  delta_flap/1 -> Cn_p0/1, Cnp_alpha/1

== system AFCSModel/Plane&Actuator/PlaneModel/Aero Moment/Calculate Yaw Moment N/aeroMoment coef/Cy_beta ==
  alpha : Inport
  Ma : Inport  Port=2
  delta_flap : Inport  Port=3
  Add1 : Sum
  Cy_beta0 : Lookup2D  RowIndex=[0 6/57.3]  ColumnIndex=Mach_table  Table=Cybeta0  SaturateOnIntegerOverflow=off  InputSameDT=off
  Cy_beta_alpha : Lookup2D  RowIndex=[0 6/57.3]  ColumnIndex=Mach_table  Table=Cybtaf  SaturateOnIntegerOverflow=off  InputSameDT=off
  Product5 : Product  RndMeth=Zero
  Cybeta : Outport
  wires:
  Cy_beta0/1 -> Add1/1
  Cy_beta_alpha/1 -> Product5/1
  Product5/1 -> Add1/2
  Ma/1 -> Cy_beta_alpha/2, Cy_beta0/2
  Add1/1 -> Cybeta/1
  alpha/1 -> Product5/2
  delta_flap/1 -> Cy_beta0/1, Cy_beta_alpha/1

== system AFCSModel/Plane&Actuator/PlaneModel/Aero Moment/Calculate pitch Moment M/Calculate Delta_M/alpha_w_deg ==
  In1 : Inport
  Constant : Constant  Value=4
  S3 : Gain  Gain=57.3
  Subtract : Sum
  Out1 : Outport
  wires:
  S3/1 -> Subtract/1
  Constant/1 -> Subtract/2
  In1/1 -> S3/1
  Subtract/1 -> Out1/1

== matlab function AFCSModel/RNP AR Approach Guidance/L1GuidanceVersion1/guidanceL1 ==
  data: eta1 input; L1 output; YZ input; Lfw input; R_turn input; turnDir input; legType input; eta output
function [L1, eta] = L1_Guidance_Logic(eta1, YZ, Lfw, R_turn, turnDir, legType)
    % ---------------------------------------------------------------------
    % 固翼无人机 L1 非线性制导律 (完美适配 RNPAR 飞行计划解析逻辑)
    % ---------------------------------------------------------------------

    % 1. 统一计算动态 L1 距离
    L1 = sqrt(YZ^2 + Lfw^2);
    
    if legType == 0
        % =================================================================
        % 【直线段逻辑】 
        % 你的示波器显示直线段已完美收敛，这部分保持不变！
        % =================================================================
        eta = atan(YZ / Lfw) - eta1;
        
    else
        % =================================================================
        % 【圆弧段逻辑】
        % =================================================================
        
        % ★ 终极修复：完美对接你的 Para_XTK 公式！
        % 因为你的代码是 Para_XTK = turnDir * (d - R_turn)
        % 所以绝对距离 d 必须通过乘以 turnDir 还原，解决左转正反馈发散问题
        d = R_turn + YZ * turnDir; 
        
        % 防止飞机刚好飞越圆心导致除零溢出奇点
        if d < 0.1
            d = 0.1;
        end
        
        % 利用余弦定理计算夹角 alpha
        cos_alpha = (d^2 + L1^2 - R_turn^2) / (2 * d * L1);
        cos_alpha = max(min(cos_alpha, 1), -1); % 防复数安全限幅
        sin_alpha = sqrt(1 - cos_alpha^2);
        
        % 计算速度矢量与圆心矢量的夹角 beta
        beta = -eta1 + (pi/2) * turnDir;
        
        % 纯代数几何拼装 L1 视线前置角
        sin_eta = sin(beta) * cos_alpha - turnDir * cos(beta) * sin_alpha;
        
        % 安全限幅与还原
        sin_eta = max(min(sin_eta, 1), -1);
        eta = asin(sin_eta);
    end
    
    % 防溢出归一化 (Wrap to Pi)，防止角度出现 359度 - 1度 = 358度 的暴力满舵
    eta = mod(eta + pi, 2*pi) - pi;
    
end

== matlab function AFCSModel/RNP AR Approach Guidance/L1GuidanceVersion1/guidanceL2Plus ==
  data: eta1 input; L1_out output; YZ input; L2_in input; R_turn input; turnDir input; legType input; eta output
function [L1_out, eta] = L2_Guidance_Plus(eta1, YZ, L2_in, R_turn, turnDir, legType)
    % ---------------------------------------------------------------------
    % 固翼无人机 L2+ 非线性制导律 (引入大误差虚拟瞄准点)
    % ---------------------------------------------------------------------
    
    % L2+ 算法大横向误差虚拟瞄准点参数
    gamma_max = 45 * pi / 180; % 最大切入角限制 (通常为 45 度)
    M_star = 2.0;              % 顺延距离乘子系数 M*
    
    % 输入的 Lfw 在 L2+ 架构中即为设定的名义前视距离 |L2|
    L2_nom = L2_in; 

    if legType == 0
        % =================================================================
        % 【直线段逻辑 - L2+ 虚拟瞄准点】
        % =================================================================
        if abs(YZ) <= L2_nom
            % 横向误差小于名义前视距离：经典 L1 几何精确求交
            x_aim = sqrt(L2_nom^2 - YZ^2);
            L1_out = L2_nom;
        else
            % 横向误差大于名义前视距离：激活 L2+ 虚拟瞄准点
            x_max_angle = abs(YZ) / tan(gamma_max);
            x_max_dist  = M_star * L2_nom;
            
            % 取两者中较小的一个作为直线上前向顺延距离
            x_aim = min(x_max_angle, x_max_dist);
            
            % 重新计算实际有效的前视距离斜边
            L1_out = sqrt(YZ^2 + x_aim^2);
        end
        
        % 计算视线角 eta
        % atan2 可自动处理全部象限，更为稳健
        eta = atan2(YZ, x_aim) - eta1;
        
    else
        % =================================================================
        % 【圆弧段逻辑 - 引入 L2+ 等效距离扩展】
        % =================================================================
        d = R_turn + YZ * turnDir; 
        
        if d < 0.1
            d = 0.1;
        end
        
        % 采用与直线段相同的约束逻辑动态计算圆弧上的有效 L1 距离
        % 以防止远距离切入圆弧时产生数学奇点
        if abs(YZ) <= L2_nom
            L1_eff = L2_nom;
        else
            x_max_angle = abs(YZ) / tan(gamma_max);
            x_max_dist  = M_star * L2_nom;
            x_aim = min(x_max_angle, x_max_dist);
            L1_eff = sqrt(YZ^2 + x_aim^2);
        end
        
        L1_out = L1_eff;
        
        % 余弦定理求交（带有防复数限幅保护）
        cos_alpha = (d^2 + L1_eff^2 - R_turn^2) / (2 * d * L1_eff);
        cos_alpha = max(min(cos_alpha, 1), -1); 
        sin_alpha = sqrt(1 - cos_alpha^2);
        
        beta = -eta1 + (pi/2) * turnDir;
        
        sin_eta = sin(beta) * cos_alpha - turnDir * cos(beta) * sin_alpha;
        
        sin_eta = max(min(sin_eta, 1), -1);
        eta = asin(sin_eta);
    end
    
    % 防溢出归一化处理 (Wrap to Pi)
    eta = mod(eta + pi, 2*pi) - pi;
    
end
